simulink model "diagrama"  (R2014b)
settings: Solver=FixedStepDiscrete  StartTime=0.0  StopTime=Te  FixedStep=Tm  RelTol=1e-3
StopFcn:
  | salida(simout)
values from neighbouring files (symbols this model uses):
  D = 0.05    [globales.mat]
  I = 0    [globales.mat]
  Kb = 0    [globales.mat]
  P = 0.1    [globales.mat]
  Pf = 50    [globales.mat]    (also in m_CS_PIDPr.m)
  Pi = -50    [globales.mat]    (also in m_CS_PIDPr.m)
  Tm = 0.01    [globales.mat]
  Tp = 5    [globales.mat]    (also in m_CS_PIDPr.m)
undefined symbols (not defined in the file or in its folder): A, B, Humusoft, MF624
undefined symbols (not defined in the file): Fcd, Fcp, Np
libraries: rtwinlib x3
settings Model: SimulationMode=external  ExtModeTrigDuration=10000  Creator=Equipo-Servo  LastModifiedBy=E. Rubio
settings DebuggingCC: UnderspecifiedInitializationDetection=Classic  MergeDetectMultiDrivingBlocksExec=none  StateNameClashWarn=warning
settings HardwareCC: ProdIntDivRoundTo=Zero  ProdEndianess=LittleEndian  ProdHWDeviceType=Generic->32-bit x86 compatible
settings RTWCC: SystemTargetFile=rtwin.tlc  TemplateMakefile=rtwin.tmf  Description=Real-Time Windows Target  ProcessScript=rtwin_make_rtw_hook  RTWCompilerOptimization=On
settings CodeAppCC: MaxIdLength=95
settings RTWinTargetCC: TargetLibSuffix=_rtwin.lib  TargetPreCompLibLocation=C:\Program Files\MATLAB\R2014b\toolbox\rtw\targets\rtwin\lib\win64

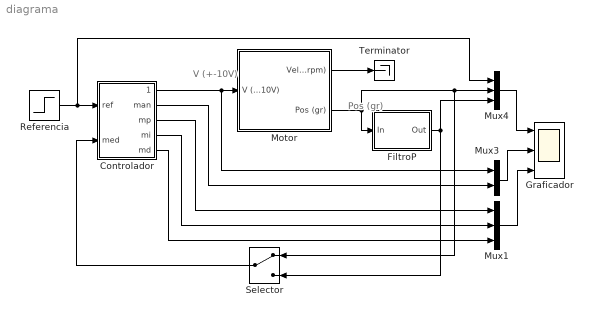
== system diagrama ==
  note: Pos
      | (gr)
  note: V (+-10V)
  Controlador : Subsystem  mask{T=Tm, P=P, I=I, Kb=Kb, D=D, Fcd=Fcd}
      mask prompts: T "Período de muestreo"; Kb "Kb (anti windup)"; Fcd "Fcd (Hz)"
      mask init:
      | N = 2*pi*Fcd;
  FiltroP : Subsystem  mask{N=Np, Fc=Fcp, Fm=1/Tm}
      mask prompts: N "Orden del filtro (Butterworth)"; Fc "Frecuencia de corte (Fc<Fm/2)"; Fm "Frecuencia de muestreo"
      mask init:
      | Fn = Fm/2;   % Frecuencia de Nyquist
      | [B,A] = butter(N,Fc/Fn);
  Graficador : Scope  NumInputPorts=3
      settings: TimeRange=10  YMin=-200~-10~-10  YMax=200~30~30  SampleTime=Tm
  Motor : Subsystem
  Mux1 : Mux  Inputs=3
  Mux3 : Mux  Inputs=2
  Mux4 : Mux  Inputs=3
  Referencia : Step  Time=Tp  Before=Pi  After=Pf  SampleTime=0
  Selector : ManualSwitch
  Terminator : Terminator
  wires:
  Mux4/1 -> Graficador/1
  Motor/2(Pos (gr)) -> Selector/1, Mux4/2, FiltroP/1(In)
  Referencia/1 -> Mux4/1, Controlador/1(ref)
  Controlador/1(mans) -> Mux3/1, Motor/1(V (+-10V))
  FiltroP/1(Out) -> Selector/2, Mux4/3
  Controlador/2(man) -> Mux3/2
  Controlador/3(mp) -> Mux1/1
  Controlador/4(mi) -> Mux1/2
  Controlador/5(md) -> Mux1/3
  Selector/1 -> Controlador/2(med)
  Mux3/1 -> Graficador/2
  Mux1/1 -> Graficador/3
  Motor/1(Vel (rpm)) -> Terminator/1

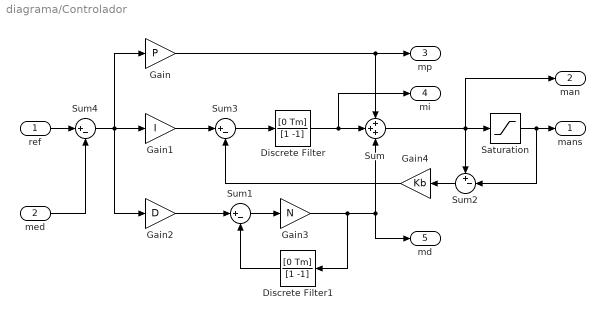
== system diagrama/Controlador ==
  ref : Inport
  med : Inport  Port=2
  Discrete Filter : DiscreteFilter  Numerator=[0 Tm]  Denominator=[1 -1]
  Discrete Filter1 : DiscreteFilter  Numerator=[0 Tm]  Denominator=[1 -1]
  Gain : Gain  Gain=P
  Gain1 : Gain  Gain=I
  Gain2 : Gain  Gain=D
  Gain3 : Gain  Gain=N
  Gain4 : Gain  Gain=Kb
  Saturation : Saturate  UpperLimit=10  LowerLimit=-10
  Sum : Sum  Inputs=+++
  Sum1 : Sum  Inputs=|+-
  Sum2 : Sum  Inputs=+-|
  Sum3 : Sum  Inputs=|+-
  Sum4 : Sum  Inputs=|+-
  mans : Outport
  man : Outport  Port=2
  mp : Outport  Port=3
  mi : Outport  Port=4
  md : Outport  Port=5
  wires:
  Sum/1 -> man/1, Sum2/1, Saturation/1
  Saturation/1 -> Sum2/2, mans/1
  Gain/1 -> Sum/1, mp/1
  Discrete Filter/1 -> mi/1, Sum/2
  ref/1 -> Sum4/1
  Sum1/1 -> Gain3/1
  Gain2/1 -> Sum1/1
  Discrete Filter1/1 -> Sum1/2
  Gain3/1 -> Discrete Filter1/1, md/1, Sum/3
  Sum2/1 -> Gain4/1
  Sum3/1 -> Discrete Filter/1
  Gain1/1 -> Sum3/1
  Gain4/1 -> Sum3/2
  Sum4/1 -> Gain2/1, Gain/1, Gain1/1
  med/1 -> Sum4/2

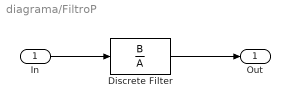
== system diagrama/FiltroP ==
  In : Inport
  Discrete Filter : DiscreteFilter  Numerator=B  Denominator=A
  Out : Outport
  wires:
  Discrete Filter/1 -> Out/1
  In/1 -> Discrete Filter/1

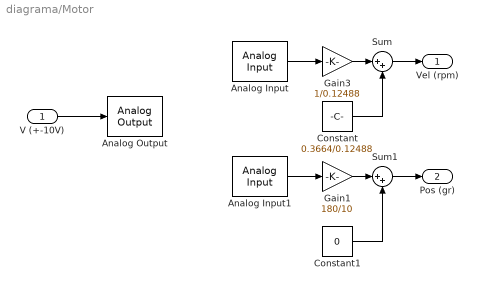
== system diagrama/Motor ==
  V (+-10V) : Inport
  Analog Input : rtwinlib/Analog Input  SampleTime=Tm  MaxMissedTicks=10  ShowMissedTicks=off  YieldWhenWaiting=off  DrvName=Humusoft/MF624  DrvAddress=0  DrvOptions=0  Channels=1  RangeMode=1  VoltRange=1  DataType=1
      settings: AttributesFormatString=Humusoft\nMF624 [0h]
  Analog Input1 : rtwinlib/Analog Input  SampleTime=Tm  MaxMissedTicks=10  ShowMissedTicks=off  YieldWhenWaiting=off  DrvName=Humusoft/MF624  DrvAddress=0  DrvOptions=0  Channels=2  RangeMode=1  VoltRange=1  DataType=1
      settings: AttributesFormatString=Humusoft\nMF624 [0h]
  Analog Output : rtwinlib/Analog Output  SampleTime=Tm  MaxMissedTicks=10  ShowMissedTicks=off  YieldWhenWaiting=off  DrvName=Humusoft/MF624  DrvAddress=0  DrvOptions=0  Channels=1  RangeMode=1  VoltRange=1  InitialValue=0  FinalValue=0
      settings: AttributesFormatString=Humusoft\nMF624 [0h]
  Constant : Constant  Value=0.3664/0.12488
  Constant1 : Constant  Value=0
  Gain1 : Gain  Gain=180/10
  Gain3 : Gain  Gain=1/0.12488
  Sum : Sum  Inputs=|++
  Sum1 : Sum  Inputs=|++
  Vel (rpm) : Outport
  Pos (gr) : Outport  Port=2
  wires:
  V (+-10V)/1 -> Analog Output/1
  Analog Input/1 -> Gain3/1
  Constant/1 -> Sum/2
  Sum/1 -> Vel (rpm)/1
  Gain3/1 -> Sum/1
  Analog Input1/1 -> Gain1/1
  Constant1/1 -> Sum1/2
  Gain1/1 -> Sum1/1
  Sum1/1 -> Pos (gr)/1
